simulink model "controller_dev_sg_RCP"  (R2018b)
settings: configuration reference "Active" (kept outside this file)
model workspace (MAT data in the model file):
  m = 1000
undefined symbols (not defined in the file or in its folder): C, tS, TUMHealthStatus, TUMVehicleState
libraries: xpcrtudplib x6, simulink x6, canmsglib x6, etargetslib x5, misc x4, speedgoatlib_IO614 x3, slrtlib x2
(part 3 of 3)

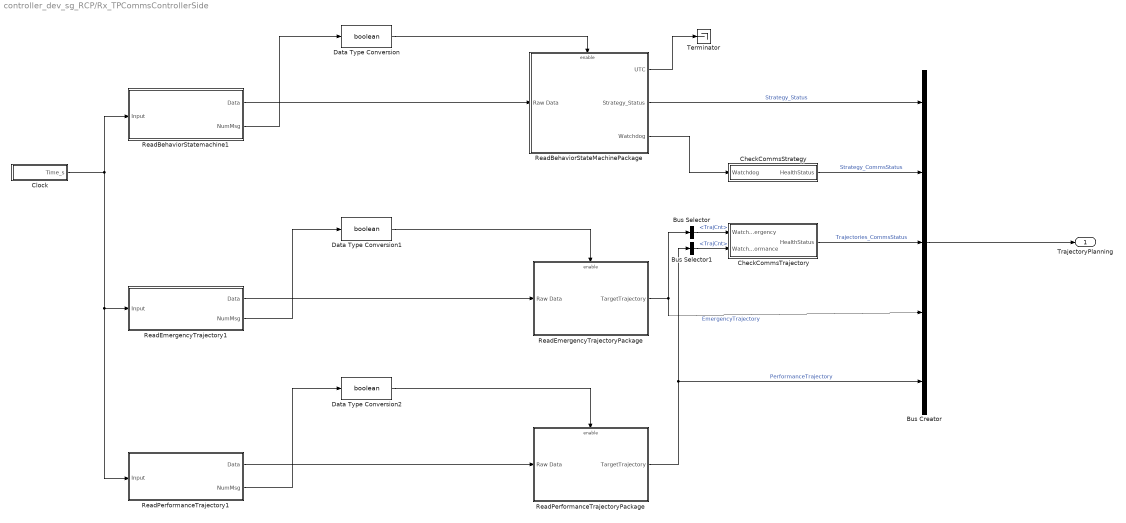
== system controller_dev_sg_RCP/Rx_TPCommsControllerSide ==
  Bus Creator : BusCreator  Inputs=5
  Bus Selector : BusSelector  OutputSignals=TrajCnt
  Bus Selector1 : BusSelector  OutputSignals=TrajCnt
  CheckCommsStrategy : Subsystem
  CheckCommsTrajectory : Subsystem
  Clock : Subsystem
  Data Type Conversion : DataTypeConversion  OutDataTypeStr=boolean
  Data Type Conversion1 : DataTypeConversion  OutDataTypeStr=boolean
  Data Type Conversion2 : DataTypeConversion  OutDataTypeStr=boolean
  ReadBehaviorStateMachinePackage : Subsystem  Priority=1000
  ReadBehaviorStatemachine1 : Subsystem  Priority=1
  ReadEmergencyTrajectory1 : Subsystem  Priority=1000
  ReadEmergencyTrajectoryPackage : Subsystem  Priority=1000
  ReadPerformanceTrajectory1 : Subsystem  Priority=1000
  ReadPerformanceTrajectoryPackage : Subsystem  Priority=1000
  Terminator : Terminator
  TrajectoryPlanning : Outport  OutDataTypeStr=Bus: TrajectoryPlanning  BusOutputAsStruct=on
  wires:
  ReadBehaviorStateMachinePackage/1(UTC) -> Terminator/1
  ReadPerformanceTrajectoryPackage/1(TargetTrajectory) -> Bus Selector1/1, Bus Creator/5  "PerformanceTrajectory"
  Clock/1(Time_s) -> ReadPerformanceTrajectory1/1(Input), ReadEmergencyTrajectory1/1(Input), ReadBehaviorStatemachine1/1(Input)
  CheckCommsTrajectory/1(HealthStatus) -> Bus Creator/3  "Trajectories_CommsStatus"
  ReadBehaviorStateMachinePackage/2(Strategy_Status) -> Bus Creator/1  "Strategy_Status"
  CheckCommsStrategy/1(HealthStatus) -> Bus Creator/2  "Strategy_CommsStatus"
  ReadEmergencyTrajectoryPackage/1(TargetTrajectory) -> Bus Selector/1, Bus Creator/4  "EmergencyTrajectory"
  Bus Selector/1 -> CheckCommsTrajectory/1(WatchdogEmergency)  "<TrajCnt>"
  Bus Selector1/1 -> CheckCommsTrajectory/2(WatchdogPerformance)  "<TrajCnt>"
  ReadBehaviorStateMachinePackage/3(Watchdog) -> CheckCommsStrategy/1(Watchdog)
  ReadEmergencyTrajectory1/2(NumMsg) -> Data Type Conversion1/1
  ReadPerformanceTrajectory1/2(NumMsg) -> Data Type Conversion2/1
  ReadBehaviorStatemachine1/2(NumMsg) -> Data Type Conversion/1
  ReadBehaviorStatemachine1/1(Data) -> ReadBehaviorStateMachinePackage/1(Raw Data)
  Data Type Conversion/1 -> ReadBehaviorStateMachinePackage/Enable
  Bus Creator/1 -> TrajectoryPlanning/1
  Data Type Conversion1/1 -> ReadEmergencyTrajectoryPackage/Enable
  ReadEmergencyTrajectory1/1(Data) -> ReadEmergencyTrajectoryPackage/1(Raw Data)
  ReadPerformanceTrajectory1/1(Data) -> ReadPerformanceTrajectoryPackage/1(Raw Data)
  Data Type Conversion2/1 -> ReadPerformanceTrajectoryPackage/Enable

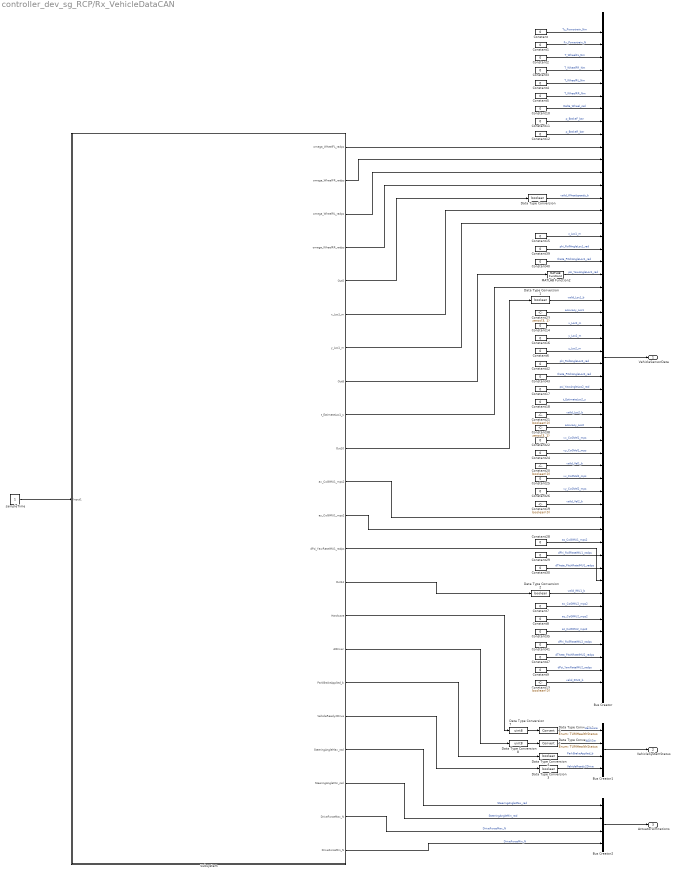
== system controller_dev_sg_RCP/Rx_VehicleDataCAN ==
  Bus Creator : BusCreator  Inputs=52  OutDataTypeStr=Bus: VehicleSensorData
  Bus Creator1 : BusCreator  Inputs=4  OutDataTypeStr=Bus: VehicleSystemStatus
  Bus Creator2 : BusCreator  Inputs=4  OutDataTypeStr=Bus: ActuatorLimitations
  Constant{,1..12,14..18,22,24..26,28..30,35,39..43,47} (32 alike) : Constant  Value=0
  Constant{13,19..21} (4 alike) : Constant  Value=boolean(0)
  Constant23 : Constant  Value=zeros(3, 1)
  Constant38 : Constant  Value=zeros(3, 1)
  Data Type Conversion{,1..4} (5 alike) : DataTypeConversion  OutDataTypeStr=boolean
  Data Type Conversion5 : DataTypeConversion  OutDataTypeStr=Enum: TUMHealthStatus
  Data Type Conversion6 : DataTypeConversion  OutDataTypeStr=Enum: TUMHealthStatus
  Data Type Conversion7 : DataTypeConversion  OutDataTypeStr=uint8
  Data Type Conversion8 : DataTypeConversion  OutDataTypeStr=uint8
  MATLAB Function2 : misc/MATLAB Function2  SystemSampleTime=-1
  Subsystem : Subsystem
  sampleTime : Constant  SampleTime=tS
  VehicleSensorData : Outport  OutDataTypeStr=Bus: VehicleSensorData
  VehicleSystemStatus : Outport  Port=2  OutDataTypeStr=Bus: VehicleSystemStatus
  ActuatorLImitations : Outport  Port=3  OutDataTypeStr=Bus: ActuatorLimitations
  wires:
  Constant30/1 -> Bus Creator/43  "dTheta_PitchRateIMU1_radps"
  Constant12/1 -> Bus Creator/9  "p_BrakeR_bar"
  Constant5/1 -> Bus Creator/6  "T_WheelRR_Nm"
  Constant1/1 -> Bus Creator/2  "Fx_Powertrain_N"
  Constant19/1 -> Bus Creator/38  "valid_Vel2_b"
  Constant7/1 -> Bus Creator/46  "ax_CoGIMU2_mps2"
  Constant11/1 -> Bus Creator/8  "p_BrakeF_bar"
  Bus Creator/1 -> VehicleSensorData/1
  Constant21/1 -> Bus Creator/31  "valid_Loc2_b"
  Constant/1 -> Bus Creator/1  "Tz_Powertrain_Nm"
  Constant25/1 -> Bus Creator/36  "vx_CoGVel2_mps"
  Constant38/1 -> Bus Creator/32  "accuracy_Loc2"
  Constant8/1 -> Bus Creator/47  "ay_CoGIMU2_mps2"
  Constant3/1 -> Bus Creator/4  "T_WheelFR_Nm"
  Constant10/1 -> Bus Creator/7  "Delta_Wheel_rad"
  Constant14/1 -> Bus Creator/24  "x_Loc2_m"
  Constant40/1 -> Bus Creator/19  "theta_PitchAngleLoc1_rad"
  Constant23/1 -> Bus Creator/23  "accuracy_Loc1"
  Constant4/1 -> Bus Creator/5  "T_WheelRL_Nm"
  Constant28/1 -> Bus Creator/41  "az_CoGIMU1_mps2"
  Constant20/1 -> Bus Creator/35  "valid_Vel1_b"
  Constant6/1 -> Bus Creator/26  "z_Loc2_m"
  Constant2/1 -> Bus Creator/3  "T_WheelFL_Nm"
  Constant39/1 -> Bus Creator/18  "phi_RollAngleLoc1_rad"
  Constant15/1 -> Bus Creator/17  "z_Loc1_m"
  Constant26/1 -> Bus Creator/37  "vy_CoGVel2_mps"
  Constant16/1 -> Bus Creator/25  "y_Loc2_m"
  MATLAB Function2/1 -> Bus Creator/20  "psi_YawAngleLoc1_rad"
  Constant42/1 -> Bus Creator/27  "phi_RollAngleLoc2_rad"
  Constant9/1 -> Bus Creator/51  "dPsi_YawRateIMU2_radps"
  Constant17/1 -> Bus Creator/29  "psi_YawAngleLoc2_rad"
  Constant24/1 -> Bus Creator/34  "vy_CoGVel1_mps"
  Constant13/1 -> Bus Creator/52  "valid_IMU2_b"
  Constant29/1 -> Bus Creator/42  "dPhi_RollRateIMU1_radps"
  Constant22/1 -> Bus Creator/33  "vx_CoGVel1_mps"
  Constant18/1 -> Bus Creator/30  "t_EstimateLoc2_s"
  Constant43/1 -> Bus Creator/28  "theta_PitchAngleLoc2_rad"
  Constant47/1 -> Bus Creator/50  "dTheta_PitchRateIMU2_radps"
  Constant41/1 -> Bus Creator/49  "dPhi_RollRateIMU2_radps"
  Constant35/1 -> Bus Creator/48  "az_CoGIMU2_mps2"
  Bus Creator1/1 -> VehicleSystemStatus/1
  Bus Creator2/1 -> ActuatorLImitations/1
  Data Type Conversion/1 -> Bus Creator/14  "valid_Wheelspeeds_b"
  Data Type Conversion1/1 -> Bus Creator/22  "valid_Loc1_b"
  Data Type Conversion2/1 -> Bus Creator/45  "valid_IMU1_b"
  Data Type Conversion3/1 -> Bus Creator1/4  "VehicleReady2Drive"
  Data Type Conversion4/1 -> Bus Creator1/3  "ParkBrakeApplied_b"
  Data Type Conversion5/1 -> Bus Creator1/2  "AIDriver"
  Data Type Conversion6/1 -> Bus Creator1/1  "Hardware"
  Data Type Conversion7/1 -> Data Type Conversion6/1
  Data Type Conversion8/1 -> Data Type Conversion5/1
  Subsystem/1(omega_WheelFL_radps) -> Bus Creator/10
  Subsystem/2(omega_WheelFR_radps) -> Bus Creator/11
  Subsystem/3(omega_WheelRL_radps) -> Bus Creator/12
  Subsystem/4(omega_WheelRR_radps) -> Bus Creator/13
  Subsystem/5(Out5) -> Data Type Conversion/1
  Subsystem/6(x_Loc1_m) -> Bus Creator/15
  Subsystem/7(y_Loc1_m) -> Bus Creator/16
  Subsystem/8(Out8) -> MATLAB Function2/1
  Subsystem/9(t_EstimateLoc1_s) -> Bus Creator/21
  Subsystem/10(Out10) -> Data Type Conversion1/1
  Subsystem/11(ax_CoGIMU1_mps2) -> Bus Creator/39
  Subsystem/12(ay_CoGIMU1_mps2) -> Bus Creator/40
  Subsystem/13(dPsi_YawRateIMU1_radps) -> Bus Creator/44
  Subsystem/14(Out14) -> Data Type Conversion2/1
  Subsystem/15(Hardware) -> Data Type Conversion7/1
  Subsystem/16(AIDriver) -> Data Type Conversion8/1
  Subsystem/17(ParkBrakeApplied_b) -> Data Type Conversion4/1
  Subsystem/18(VehicleReady2Drive) -> Data Type Conversion3/1
  sampleTime/1 -> Subsystem/1(Input1)
  Subsystem/22(DriveForceMin_N) -> Bus Creator2/4  "DriveForceMin_N"
  Subsystem/19(SteeringAngleMax_rad) -> Bus Creator2/1  "SteeringAngleMax_rad"
  Subsystem/20(SteeringAngleMin_rad) -> Bus Creator2/2  "SteeringAngleMin_rad"
  Subsystem/21(DriveForceMax_N) -> Bus Creator2/3  "DriveForceMax_N"

== system controller_dev_sg_RCP/Tx_TPCommsControllerSide ==
  VehicleDynamicState : Inport
  TrajPlannerSend : Inport  Port=2
  DebugData : Inport  Port=3
  BehaviorStatemachine : Subsystem
  Digital Clock : DigitalClock  SampleTime=-1
  SendToBehaviorStatemachine1 : Subsystem
  SendToTrajectoryGeneration1 : Subsystem
  TrajectoryGeneration : Subsystem
  wires:
  DebugData/1 -> BehaviorStatemachine/2(DebugData)
  TrajPlannerSend/1 -> TrajectoryGeneration/1(TrajPlannerSend), BehaviorStatemachine/1(TrajPlannerSend)
  VehicleDynamicState/1 -> TrajectoryGeneration/2(VehicleDynamicState)
  Digital Clock/1 -> TrajectoryGeneration/3(Time_s)
  BehaviorStatemachine/2(BSM_Package) -> SendToBehaviorStatemachine1/1(Data)  "BSM_Package"
  TrajectoryGeneration/2(TG_Package) -> SendToTrajectoryGeneration1/1(Data)
  TrajectoryGeneration/1(TG_ActivateSend) -> SendToTrajectoryGeneration1/Enable  "TG_ActivateSend"
  BehaviorStatemachine/1(BSM_ActivateSend) -> SendToBehaviorStatemachine1/Enable  "BSM_ActivateSend"

== system controller_dev_sg_RCP/Tx_VehicleControlCAN ==
  SteeringAngleAtWheel_rad : Inport
  TractionForceSummedAtWheels_N : Inport  Port=2
  "CAN Pack " : canmsglib/CAN Pack  MsgList=(none)  MsgName=CAN Msg  MsgIDType=Standard (11-bit identifier)  MsgIdentifier=24  MsgLength=8  SignalInfo=SteeringAngleAtWheel_rad$0$24$1$1$1$0$0.000001$0$-Inf$Inf$#TractionForceSummedAtWheels_N$24$24$1$1$1$0$0.01$0$-Inf$Inf$#  NSignals=2  StartBits=str2num('[int32(0);int32(24)]')  SignalSizes=str2num('[int32(24);int32(24)]')  ByteOrders=str2num('[int32(1);int32(1)]')  DataTypes=str2num('[int32(1);int32(1)]')  MultiplexTypes=str2num('[int32(1);int32(1)]')  MultiplexValues=str2num('[double(0);double(0)]')  Factors=str2num('[double(0.000001);double(0.01)]')  Offsets=str2num('[double(0);double(0)]')  Minimums=str2num('[double(-Inf);double(-Inf)]')  Maximums=str2num('[double(Inf);double(Inf)]')  Remote=off  ApplyMinMax=off  BusOutput=off
      settings: SourceProductName=Simulink Real-Time  DataFormat=manually specified signals
  CAN Write : speedgoatlib_IO614/CAN/CAN Write  id=1  sampleTime=-1  portSelection=2  messageType=CAN  enaStatusPort=off  protl=IO614  ptIdx=1  isFDMod=0
      settings: SourceProductName=Simulink Real-Time: Speedgoat Library
  wires:
  "CAN Pack "/1 -> CAN Write/1
  TractionForceSummedAtWheels_N/1 -> "CAN Pack "/2
  SteeringAngleAtWheel_rad/1 -> "CAN Pack "/1

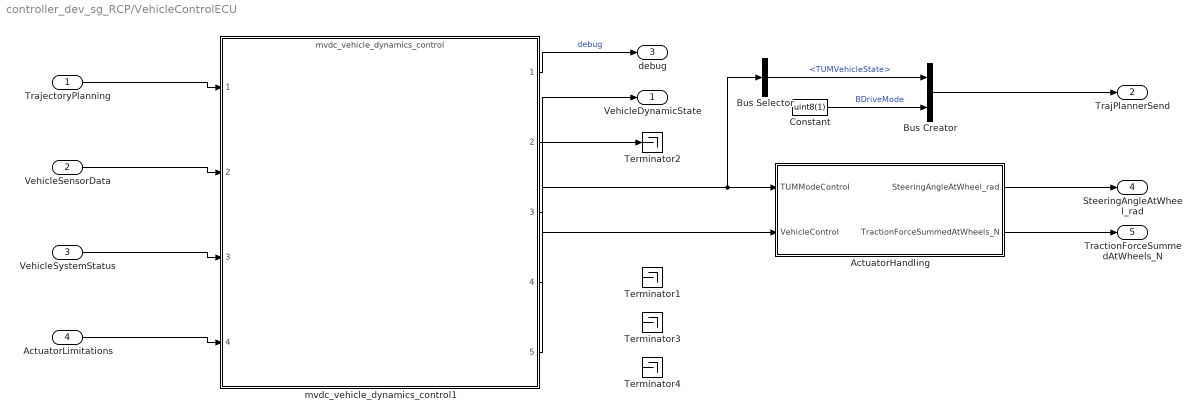
== system controller_dev_sg_RCP/VehicleControlECU ==
  TrajectoryPlanning : Inport
  VehicleSensorData : Inport  Port=2
  VehicleSystemStatus : Inport  Port=3
  ActuatorLimitations : Inport  Port=4
  ActuatorHandling : Subsystem
  Bus Creator : BusCreator  Inputs=2
  Bus Selector : BusSelector  OutputSignals=TUMVehicleState
  Constant : Constant  Value=uint8(1)
  Terminator{1..4} (4 alike) : Terminator
  mvdc_vehicle_dynamics_control1 : ModelReference  ModelNameDialog=mvdc_vehicle_dynamics_control  SimulationMode=Normal  ModelReferenceVersion=1.767
  VehicleDynamicState : Outport
  TrajPlannerSend : Outport  Port=2
  debug : Outport  Port=3
  SteeringAngleAtWheel_rad : Outport  Port=4
  TractionForceSummedAtWheels_N : Outport  Port=5
  wires:
  mvdc_vehicle_dynamics_control1/1 -> debug/1  "debug"
  VehicleSystemStatus/1 -> mvdc_vehicle_dynamics_control1/3
  ActuatorLimitations/1 -> mvdc_vehicle_dynamics_control1/4
  VehicleSensorData/1 -> mvdc_vehicle_dynamics_control1/2
  mvdc_vehicle_dynamics_control1/5 -> ActuatorHandling/2(VehicleControl)
  mvdc_vehicle_dynamics_control1/4 -> Bus Selector/1, ActuatorHandling/1(TUMModeControl)
  ? -> Terminator1/1
  mvdc_vehicle_dynamics_control1/3 -> Terminator2/1
  mvdc_vehicle_dynamics_control1/2 -> VehicleDynamicState/1
  ActuatorHandling/2(TractionForceSummedAtWheels_N) -> TractionForceSummedAtWheels_N/1
  ActuatorHandling/1(SteeringAngleAtWheel_rad) -> SteeringAngleAtWheel_rad/1
  ? -> Terminator3/1
  ? -> Terminator4/1
  Bus Selector/1 -> Bus Creator/1  "<TUMVehicleState>"
  Constant/1 -> Bus Creator/2  "BDriveMode"
  Bus Creator/1 -> TrajPlannerSend/1
  TrajectoryPlanning/1 -> mvdc_vehicle_dynamics_control1/1

== system controller_dev_sg_RCP/Rx_TPCommsControllerSide/CheckCommsStrategy ==
  Watchdog : Inport
  CheckComms : misc/CheckComms  timeout_s=tPX2CommsTimeout  tS=tS
  Constant1 : Constant  Value=TUMHealthStatus.ERROR  OutDataTypeStr=Enum: TUMHealthStatus
  Constant2 : Constant  Value=TUMHealthStatus.OK  OutDataTypeStr=Enum: TUMHealthStatus
  Switch1 : Switch  Criteria=u2 > Threshold
  HealthStatus : Outport
  wires:
  CheckComms/1 -> Switch1/2
  Constant2/1 -> Switch1/1
  Switch1/1 -> HealthStatus/1  "Strategy_CommsStatus"
  Constant1/1 -> Switch1/3
  Watchdog/1 -> CheckComms/1

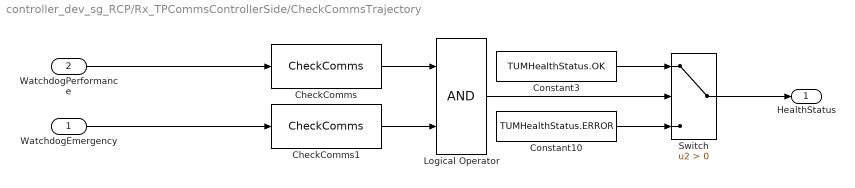
== system controller_dev_sg_RCP/Rx_TPCommsControllerSide/CheckCommsTrajectory ==
  WatchdogEmergency : Inport
  WatchdogPerformance : Inport  Port=2
  CheckComms : misc/CheckComms  timeout_s=tPX2CommsTimeout  tS=tS
  CheckComms1 : misc/CheckComms  timeout_s=tPX2CommsTimeout  tS=tS
  Constant10 : Constant  Value=TUMHealthStatus.ERROR  OutDataTypeStr=Enum: TUMHealthStatus  SampleTime=-1
  Constant3 : Constant  Value=TUMHealthStatus.OK  OutDataTypeStr=Enum: TUMHealthStatus  SampleTime=-1
  Logical Operator : Logic  AllPortsSameDT=off  OutDataTypeStr=boolean
  Switch : Switch  Criteria=u2 > Threshold
  HealthStatus : Outport
  wires:
  Constant10/1 -> Switch/3
  Logical Operator/1 -> Switch/2
  CheckComms/1 -> Logical Operator/1
  CheckComms1/1 -> Logical Operator/2
  Constant3/1 -> Switch/1
  Switch/1 -> HealthStatus/1
  WatchdogEmergency/1 -> CheckComms1/1
  WatchdogPerformance/1 -> CheckComms/1

== system controller_dev_sg_RCP/Rx_TPCommsControllerSide/Clock ==
  Counter Free-Running : simulink/Sources/Counter Free-Running  NumBits=32  tsamp=tS
  Data Type Conversion : DataTypeConversion  OutDataTypeStr=double  SaturateOnIntegerOverflow=on
  Gain : Gain  Gain=tS
  Time_s : Outport
  wires:
  Counter Free-Running/1 -> Data Type Conversion/1
  Gain/1 -> Time_s/1
  Data Type Conversion/1 -> Gain/1

== system controller_dev_sg_RCP/Rx_TPCommsControllerSide/ReadBehaviorStateMachinePackage ==
  Raw Data : Inport
  Enable : EnablePort
  Byte Unpack : etargetslib/Byte Unpack  dimensions={[1], [1], [1]}  datatypes={'uint16', 'uint16', 'uint32'}  byteAlign=1
  Data Type Conversion : DataTypeConversion  OutDataTypeStr=Enum: TUMStrategyState  SaturateOnIntegerOverflow=on
  UTC : Outport
  Strategy_Status : Outport  Port=2  OutDataTypeStr=Enum: TUMStrategyState
  Watchdog : Outport  Port=3
  wires:
  Byte Unpack/1 -> Data Type Conversion/1
  Data Type Conversion/1 -> Strategy_Status/1
  Byte Unpack/2 -> Watchdog/1
  Raw Data/1 -> Byte Unpack/1
  Byte Unpack/3 -> UTC/1

== system controller_dev_sg_RCP/Rx_TPCommsControllerSide/ReadBehaviorStatemachine1 ==
  Input : Inport
  Compare To Constant : simulink/Logic and Bit Operations/Compare To Constant  Priority=1  relop===  const=8  OutDataTypeStr=boolean
  Min. do-while count : Constant  OutDataTypeStr=int8  SampleTime=-1
  Subtrat : Sum  Inputs=+-
  Terminator : Terminator
  UDP Receive : xpcrtudplib/UDP Receive  ipAddressVal=10.0.0.1  localPort=BehaviorStatemachineRcv_Port  rcvWidth=8  rcvFmAny=off  fmAddress=10.0.0.2  rcvMulticast=off  multicastAddress={}  maxUDPQueue=8  sampleTime=-1
      settings: SourceProductName=Simulink Real-Time
  While Iterator : WhileIterator  WhileBlockType=do-while  ShowIterationPort=on  OutputDataType=int16
  Data : Outport
  NumMsg : Outport  Port=2
  wires:
  Compare To Constant/1 -> While Iterator/1
  UDP Receive/2 -> Compare To Constant/1
  While Iterator/1 -> Subtrat/1
  Min. do-while count/1 -> Subtrat/2
  UDP Receive/1 -> Data/1
  Subtrat/1 -> NumMsg/1  "num msgs this timestep"
  Input/1 -> Terminator/1

== system controller_dev_sg_RCP/Rx_TPCommsControllerSide/ReadEmergencyTrajectory1 ==
  Input : Inport
  Compare To Constant : simulink/Logic and Bit Operations/Compare To Constant  relop===  const=4*7*50+2*4  OutDataTypeStr=boolean
  Min. do-while count : Constant  OutDataTypeStr=int8  SampleTime=-1
  Subtrat : Sum  Inputs=+-
  Terminator : Terminator
  UDP Receive : xpcrtudplib/UDP Receive  ipAddressVal=10.0.0.1  localPort=EmergencyPathRcv_Port  rcvWidth=4*7*50+2*4  rcvFmAny=off  fmAddress=10.0.0.2  rcvMulticast=off  multicastAddress={}  maxUDPQueue=8  sampleTime=-1
      settings: SourceProductName=Simulink Real-Time
  While Iterator : WhileIterator  WhileBlockType=do-while  ShowIterationPort=on  OutputDataType=int16
  Data : Outport
  NumMsg : Outport  Port=2
  wires:
  UDP Receive/2 -> Compare To Constant/1
  While Iterator/1 -> Subtrat/1
  Min. do-while count/1 -> Subtrat/2
  UDP Receive/1 -> Data/1
  Compare To Constant/1 -> While Iterator/1
  Subtrat/1 -> NumMsg/1  "num msgs this timestep"
  Input/1 -> Terminator/1

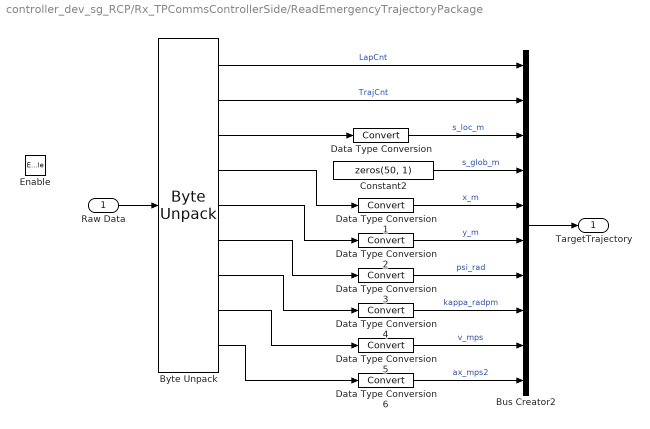
== system controller_dev_sg_RCP/Rx_TPCommsControllerSide/ReadEmergencyTrajectoryPackage ==
  Raw Data : Inport
  Enable : EnablePort
  Bus Creator2 : BusCreator  Inputs=10  OutDataTypeStr=Bus: Trajectory
      settings: InheritFromInputs=off
  Byte Unpack : etargetslib/Byte Unpack  dimensions={[1], [1], [50], [50], [50], [50], [50], [50],[50]}  datatypes={'uint32', 'uint32', 'single', 'single', 'single', 'single', 'single', 'single', 'single'}  byteAlign=1
  Constant2 : Constant  Value=zeros(50, 1)
  Data Type Conversion{,1..6} (7 alike) : DataTypeConversion
  TargetTrajectory : Outport  OutDataTypeStr=Bus: Trajectory
  wires:
  Byte Unpack/1 -> Bus Creator2/1  "LapCnt"
  Byte Unpack/2 -> Bus Creator2/2  "TrajCnt"
  Bus Creator2/1 -> TargetTrajectory/1
  Raw Data/1 -> Byte Unpack/1
  Byte Unpack/3 -> Data Type Conversion/1
  Byte Unpack/4 -> Data Type Conversion1/1
  Constant2/1 -> Bus Creator2/4  "s_glob_m"
  Data Type Conversion/1 -> Bus Creator2/3  "s_loc_m"
  Data Type Conversion1/1 -> Bus Creator2/5  "x_m"
  Data Type Conversion2/1 -> Bus Creator2/6  "y_m"
  Byte Unpack/5 -> Data Type Conversion2/1
  Data Type Conversion3/1 -> Bus Creator2/7  "psi_rad"
  Data Type Conversion4/1 -> Bus Creator2/8  "kappa_radpm"
  Data Type Conversion5/1 -> Bus Creator2/9  "v_mps"
  Data Type Conversion6/1 -> Bus Creator2/10  "ax_mps2"
  Byte Unpack/6 -> Data Type Conversion3/1
  Byte Unpack/7 -> Data Type Conversion4/1
  Byte Unpack/8 -> Data Type Conversion5/1
  Byte Unpack/9 -> Data Type Conversion6/1

== system controller_dev_sg_RCP/Rx_TPCommsControllerSide/ReadPerformanceTrajectory1 ==
  Input : Inport
  Compare To Constant : simulink/Logic and Bit Operations/Compare To Constant  relop===  const=4*7*50+2*4  OutDataTypeStr=boolean
  Min. do-while count : Constant  OutDataTypeStr=int8  SampleTime=-1
  Subtrat : Sum  Inputs=+-
  Terminator : Terminator
  UDP Receive : xpcrtudplib/UDP Receive  ipAddressVal=10.0.0.1  localPort=PerformanceTrajectoryRcv_Port  rcvWidth=4*7*50+2*4  rcvFmAny=off  fmAddress=10.0.0.2  rcvMulticast=off  multicastAddress={}  maxUDPQueue=8  sampleTime=-1
      settings: SourceProductName=Simulink Real-Time
  While Iterator : WhileIterator  WhileBlockType=do-while  ShowIterationPort=on  OutputDataType=int16
  Data : Outport
  NumMsg : Outport  Port=2
  wires:
  Compare To Constant/1 -> While Iterator/1
  UDP Receive/2 -> Compare To Constant/1
  UDP Receive/1 -> Data/1
  While Iterator/1 -> Subtrat/1
  Min. do-while count/1 -> Subtrat/2
  Subtrat/1 -> NumMsg/1  "num msgs this timestep"
  Input/1 -> Terminator/1

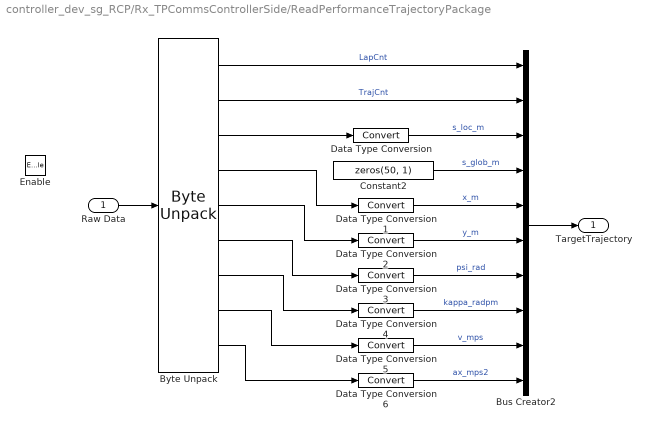
== system controller_dev_sg_RCP/Rx_TPCommsControllerSide/ReadPerformanceTrajectoryPackage ==
  Raw Data : Inport
  Enable : EnablePort
  Bus Creator2 : BusCreator  Inputs=10  OutDataTypeStr=Bus: Trajectory
      settings: InheritFromInputs=off
  Byte Unpack : etargetslib/Byte Unpack  dimensions={[1], [1], [50], [50], [50], [50], [50], [50],[50]}  datatypes={'uint32', 'uint32', 'single', 'single', 'single', 'single', 'single', 'single', 'single'}  byteAlign=1
  Constant2 : Constant  Value=zeros(50, 1)
  Data Type Conversion{,1..6} (7 alike) : DataTypeConversion
  TargetTrajectory : Outport  OutDataTypeStr=Bus: Trajectory
  wires:
  Byte Unpack/1 -> Bus Creator2/1  "LapCnt"
  Byte Unpack/2 -> Bus Creator2/2  "TrajCnt"
  Bus Creator2/1 -> TargetTrajectory/1
  Raw Data/1 -> Byte Unpack/1
  Byte Unpack/3 -> Data Type Conversion/1
  Byte Unpack/4 -> Data Type Conversion1/1
  Constant2/1 -> Bus Creator2/4  "s_glob_m"
  Data Type Conversion/1 -> Bus Creator2/3  "s_loc_m"
  Data Type Conversion1/1 -> Bus Creator2/5  "x_m"
  Data Type Conversion2/1 -> Bus Creator2/6  "y_m"
  Byte Unpack/5 -> Data Type Conversion2/1
  Data Type Conversion3/1 -> Bus Creator2/7  "psi_rad"
  Data Type Conversion4/1 -> Bus Creator2/8  "kappa_radpm"
  Data Type Conversion5/1 -> Bus Creator2/9  "v_mps"
  Data Type Conversion6/1 -> Bus Creator2/10  "ax_mps2"
  Byte Unpack/6 -> Data Type Conversion3/1
  Byte Unpack/7 -> Data Type Conversion4/1
  Byte Unpack/8 -> Data Type Conversion5/1
  Byte Unpack/9 -> Data Type Conversion6/1

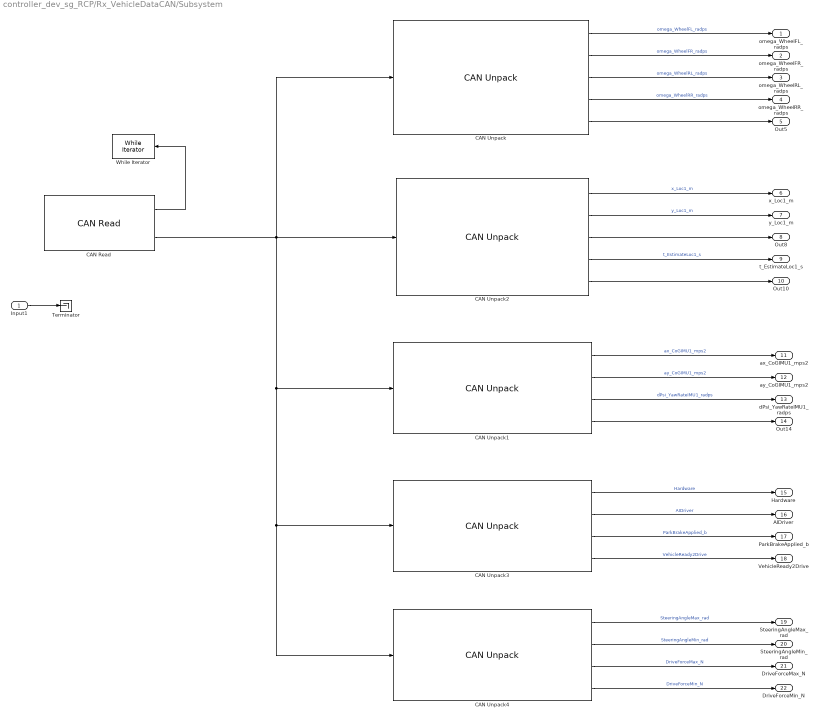
== system controller_dev_sg_RCP/Rx_VehicleDataCAN/Subsystem ==
  Input1 : Inport
  CAN Read : speedgoatlib_IO614/CAN/CAN Read  id=1  sampleTime=-1  portSelection=1  messageType=CAN  protl=IO614  ptIdx=0  isFDMod=0
      settings: SourceProductName=Simulink Real-Time: Speedgoat Library
  CAN Unpack : canmsglib/CAN Unpack  MsgList=(none)  MsgName=CAN Msg  MsgIDType=Standard (11-bit identifier)  MsgIdentifier=768  MsgLength=8  SignalInfo=omega_WheelFL_radps$0$15$1$1$1$0$0.1$0$-Inf$Inf$#omega_WheelFR_radps$15$15$1$1$1$0$0.1$0$-Inf$Inf$#omega_WheelRL_radps$30$15$1$1$1$0$0.1$0$-Inf$Inf$#omega_WheelRR_radps$45$15$1$1$1$0$0.1$0$-Inf$Inf$#valid_Wheelspeeds_b$60$4$1$1$1$0$1$0$-Inf$Inf$#  NSignals=5  IDPort=off  TimestampPort=off  ErrorPort=off  RemotePort=off  LengthPort=off  StatusPort=off  StartBits=str2num('[int32(0);int32(15);int32(30);int32(45);int32(60)]')  SignalSizes=str2num('[int32(15);int32(15);int32(15);int32(15);int32(4)]')  ByteOrders=str2num('[int32(1);int32(1);int32(1);int32(1);int32(1)]')  DataTypes=str2num('[int32(1);int32(1);int32(1);int32(1);int32(1)]')  MultiplexTypes=str2num('[int32(1);int32(1);int32(1);int32(1);int32(1)]')  MultiplexValues=str2num('[double(0);double(0);double(0);double(0);double(0)]')  Factors=str2num('[double(0.1);double(0.1);double(0.1);double(0.1);double(1)]')  Offsets=str2num('[double(0);double(0);double(0);double(0);double(0)]')  Minimums=str2num('[double(-Inf);double(-Inf);double(-Inf);double(-Inf);double(-Inf)]')  Maximums=str2num('[double(Inf);double(Inf);double(Inf);double(Inf);double(Inf)]')  ApplyMinMax=off
      settings: SourceProductName=Simulink Real-Time
  CAN Unpack1 : canmsglib/CAN Unpack  MsgList=(none)  MsgName=CAN Msg  MsgIDType=Standard (11-bit identifier)  MsgIdentifier=48  MsgLength=8  SignalInfo=ax_CoGIMU1_mps2$0$16$1$1$1$0$0.001$0$-Inf$Inf$#ay_CoGIMU1_mps2$16$16$1$1$1$0$0.001$0$-Inf$Inf$#dPsi_YawRateIMU1_radps$32$16$1$1$1$0$0.0001$0$-Inf$Inf$#valid_IMU1_b$48$16$1$1$1$0$1$0$-Inf$Inf$#  NSignals=4  IDPort=off  TimestampPort=off  ErrorPort=off  RemotePort=off  LengthPort=off  StatusPort=off  StartBits=str2num('[int32(0);int32(16);int32(32);int32(48)]')  SignalSizes=str2num('[int32(16);int32(16);int32(16);int32(16)]')  ByteOrders=str2num('[int32(1);int32(1);int32(1);int32(1)]')  DataTypes=str2num('[int32(1);int32(1);int32(1);int32(1)]')  MultiplexTypes=str2num('[int32(1);int32(1);int32(1);int32(1)]')  MultiplexValues=str2num('[double(0);double(0);double(0);double(0)]')  Factors=str2num('[double(0.001);double(0.001);double(0.0001);double(1)]')  Offsets=str2num('[double(0);double(0);double(0);double(0)]')  Minimums=str2num('[double(-Inf);double(-Inf);double(-Inf);double(-Inf)]')  Maximums=str2num('[double(Inf);double(Inf);double(Inf);double(Inf)]')  ApplyMinMax=off
      settings: SourceProductName=Simulink Real-Time
  CAN Unpack2 : canmsglib/CAN Unpack  MsgList=(none)  MsgName=CAN Msg  MsgIDType=Standard (11-bit identifier)  MsgIdentifier=192  MsgLength=8  SignalInfo=x_Loc1_m$0$15$1$1$1$0$0.05$0$-Inf$Inf$#y_Loc1_m$15$15$1$1$1$0$0.05$0$-Inf$Inf$#psi_YawAngleLoc1_rad$30$15$1$1$1$0$0.001$0$-Inf$Inf$#t_EstimateLoc1_s$45$15$1$1$1$0$0.001$0$-Inf$Inf$#valid_Loc1_b$60$4$1$1$1$0$1$0$-Inf$Inf$#  NSignals=5  IDPort=off  TimestampPort=off  ErrorPort=off  RemotePort=off  LengthPort=off  StatusPort=off  StartBits=str2num('[int32(0);int32(15);int32(30);int32(45);int32(60)]')  SignalSizes=str2num('[int32(15);int32(15);int32(15);int32(15);int32(4)]')  ByteOrders=str2num('[int32(1);int32(1);int32(1);int32(1);int32(1)]')  DataTypes=str2num('[int32(1);int32(1);int32(1);int32(1);int32(1)]')  MultiplexTypes=str2num('[int32(1);int32(1);int32(1);int32(1);int32(1)]')  MultiplexValues=str2num('[double(0);double(0);double(0);double(0);double(0)]')  Factors=str2num('[double(0.05);double(0.05);double(0.001);double(0.001);double(1)]')  Offsets=str2num('[double(0);double(0);double(0);double(0);double(0)]')  Minimums=str2num('[double(-Inf);double(-Inf);double(-Inf);double(-Inf);double(-Inf)]')  Maximums=str2num('[double(Inf);double(Inf);double(Inf);double(Inf);double(Inf)]')  ApplyMinMax=off
      settings: SourceProductName=Simulink Real-Time
  CAN Unpack3 : canmsglib/CAN Unpack  MsgList=(none)  MsgName=CAN Msg  MsgIDType=Standard (11-bit identifier)  MsgIdentifier=12  MsgLength=8  SignalInfo=Hardware$0$12$1$2$1$0$1$0$-Inf$Inf$#AIDriver$12$12$1$2$1$0$1$0$-Inf$Inf$#ParkBrakeApplied_b$24$12$1$1$1$0$1$0$-Inf$Inf$#VehicleReady2Drive$36$12$1$1$1$0$1$0$-Inf$Inf$#  NSignals=4  IDPort=off  TimestampPort=off  ErrorPort=off  RemotePort=off  LengthPort=off  StatusPort=off  StartBits=str2num('[int32(0);int32(12);int32(24);int32(36)]')  SignalSizes=str2num('[int32(12);int32(12);int32(12);int32(12)]')  ByteOrders=str2num('[int32(1);int32(1);int32(1);int32(1)]')  DataTypes=str2num('[int32(2);int32(2);int32(1);int32(1)]')  MultiplexTypes=str2num('[int32(1);int32(1);int32(1);int32(1)]')  MultiplexValues=str2num('[double(0);double(0);double(0);double(0)]')  Factors=str2num('[double(1);double(1);double(1);double(1)]')  Offsets=str2num('[double(0);double(0);double(0);double(0)]')  Minimums=str2num('[double(-Inf);double(-Inf);double(-Inf);double(-Inf)]')  Maximums=str2num('[double(Inf);double(Inf);double(Inf);double(Inf)]')  ApplyMinMax=off
      settings: SourceProductName=Simulink Real-Time
  CAN Unpack4 : canmsglib/CAN Unpack  MsgList=(none)  MsgName=CAN Msg  MsgIDType=Standard (11-bit identifier)  MsgIdentifier=170  MsgLength=8  SignalInfo=SteeringAngleMax_rad$0$16$1$1$1$0$0.001$0$-Inf$Inf$#SteeringAngleMin_rad$16$16$1$1$1$0$0.001$0$-Inf$Inf$#DriveForceMax_N$32$16$1$1$1$0$100$0$-Inf$Inf$#DriveForceMin_N$48$16$1$1$1$0$100$0$-Inf$Inf$#  NSignals=4  IDPort=off  TimestampPort=off  ErrorPort=off  RemotePort=off  LengthPort=off  StatusPort=off  StartBits=str2num('[int32(0);int32(16);int32(32);int32(48)]')  SignalSizes=str2num('[int32(16);int32(16);int32(16);int32(16)]')  ByteOrders=str2num('[int32(1);int32(1);int32(1);int32(1)]')  DataTypes=str2num('[int32(1);int32(1);int32(1);int32(1)]')  MultiplexTypes=str2num('[int32(1);int32(1);int32(1);int32(1)]')  MultiplexValues=str2num('[double(0);double(0);double(0);double(0)]')  Factors=str2num('[double(0.001);double(0.001);double(100);double(100)]')  Offsets=str2num('[double(0);double(0);double(0);double(0)]')  Minimums=str2num('[double(-Inf);double(-Inf);double(-Inf);double(-Inf)]')  Maximums=str2num('[double(Inf);double(Inf);double(Inf);double(Inf)]')  ApplyMinMax=off
      settings: SourceProductName=Simulink Real-Time
  Terminator : Terminator
  While Iterator : WhileIterator  MaxIters=501  WhileBlockType=do-while
  omega_WheelFL_radps : Outport
  omega_WheelFR_radps : Outport  Port=2
  omega_WheelRL_radps : Outport  Port=3
  omega_WheelRR_radps : Outport  Port=4
  Out5 : Outport  Port=5
  x_Loc1_m : Outport  Port=6
  y_Loc1_m : Outport  Port=7
  Out8 : Outport  Port=8
  t_EstimateLoc1_s : Outport  Port=9
  Out10 : Outport  Port=10
  ax_CoGIMU1_mps2 : Outport  Port=11
  ay_CoGIMU1_mps2 : Outport  Port=12
  dPsi_YawRateIMU1_radps : Outport  Port=13
  Out14 : Outport  Port=14
  Hardware : Outport  Port=15
  AIDriver : Outport  Port=16
  ParkBrakeApplied_b : Outport  Port=17
  VehicleReady2Drive : Outport  Port=18
  SteeringAngleMax_rad : Outport  Port=19
  SteeringAngleMin_rad : Outport  Port=20
  DriveForceMax_N : Outport  Port=21
  DriveForceMin_N : Outport  Port=22
  wires:
  CAN Read/2 -> CAN Unpack/1, CAN Unpack2/1, CAN Unpack1/1, CAN Unpack3/1, CAN Unpack4/1
  CAN Unpack/4 -> omega_WheelRR_radps/1  "omega_WheelRR_radps"
  CAN Unpack2/2 -> y_Loc1_m/1  "y_Loc1_m"
  CAN Unpack2/5 -> Out10/1
  Input1/1 -> Terminator/1
  CAN Unpack/5 -> Out5/1
  CAN Read/1 -> While Iterator/1
  CAN Unpack1/1 -> ax_CoGIMU1_mps2/1  "ax_CoGIMU1_mps2"
  CAN Unpack2/4 -> t_EstimateLoc1_s/1  "t_EstimateLoc1_s"
  CAN Unpack2/3 -> Out8/1
  CAN Unpack/1 -> omega_WheelFL_radps/1  "omega_WheelFL_radps"
  CAN Unpack4/3 -> DriveForceMax_N/1  "DriveForceMax_N"
  CAN Unpack/3 -> omega_WheelRL_radps/1  "omega_WheelRL_radps"
  CAN Unpack1/2 -> ay_CoGIMU1_mps2/1  "ay_CoGIMU1_mps2"
  CAN Unpack4/2 -> SteeringAngleMin_rad/1  "SteeringAngleMin_rad"
  CAN Unpack3/2 -> AIDriver/1  "AIDriver"
  CAN Unpack3/3 -> ParkBrakeApplied_b/1  "ParkBrakeApplied_b"
  CAN Unpack1/4 -> Out14/1
  CAN Unpack4/1 -> SteeringAngleMax_rad/1  "SteeringAngleMax_rad"
  CAN Unpack/2 -> omega_WheelFR_radps/1  "omega_WheelFR_radps"
  CAN Unpack2/1 -> x_Loc1_m/1  "x_Loc1_m"
  CAN Unpack3/4 -> VehicleReady2Drive/1  "VehicleReady2Drive"
  CAN Unpack3/1 -> Hardware/1  "Hardware"
  CAN Unpack1/3 -> dPsi_YawRateIMU1_radps/1  "dPsi_YawRateIMU1_radps"
  CAN Unpack4/4 -> DriveForceMin_N/1  "DriveForceMin_N"

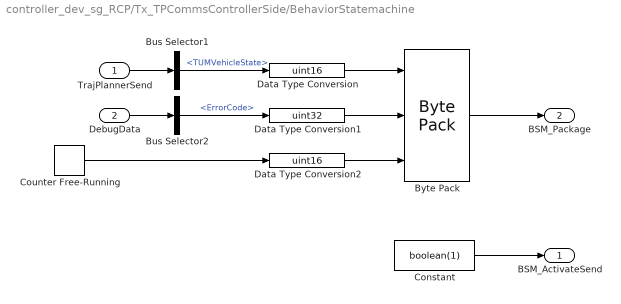
== system controller_dev_sg_RCP/Tx_TPCommsControllerSide/BehaviorStatemachine ==
  TrajPlannerSend : Inport
  DebugData : Inport  Port=2  OutDataTypeStr=Bus: mvdc_vehicle_dynamics_control_debug  PortDimensions=1
  Bus Selector1 : BusSelector  OutputSignals=TUMVehicleState
  Bus Selector2 : BusSelector  OutputSignals=ErrorCode
  Byte Pack : etargetslib/Byte Pack  datatypes={'uint16', 'uint32', 'uint16'}  byteAlign=1
  Constant : Constant  Value=boolean(1)  SampleTime=-1
  Counter Free-Running : simulink/Sources/Counter Free-Running  NumBits=8  tsamp=-1
  Data Type Conversion : DataTypeConversion  OutDataTypeStr=uint16
  Data Type Conversion1 : DataTypeConversion  OutDataTypeStr=uint32
  Data Type Conversion2 : DataTypeConversion  OutDataTypeStr=uint16
  BSM_ActivateSend : Outport
  BSM_Package : Outport  Port=2
  wires:
  Counter Free-Running/1 -> Data Type Conversion2/1
  Data Type Conversion/1 -> Byte Pack/1
  Data Type Conversion2/1 -> Byte Pack/3
  Byte Pack/1 -> BSM_Package/1
  Constant/1 -> BSM_ActivateSend/1
  TrajPlannerSend/1 -> Bus Selector1/1
  Bus Selector1/1 -> Data Type Conversion/1  "<TUMVehicleState>"
  DebugData/1 -> Bus Selector2/1
  Bus Selector2/1 -> Data Type Conversion1/1  "<ErrorCode>"
  Data Type Conversion1/1 -> Byte Pack/2

== system controller_dev_sg_RCP/Tx_TPCommsControllerSide/SendToBehaviorStatemachine1 ==
  Data : Inport
  Enable : EnablePort
  "Send " : xpcrtudplib/UDP Send  ipAddressVal=10.0.0.1  localPort=-1  toAddress=10.0.0.2  toPort=BehaviorStatemachineSend_Port  sampleTime=-1
      settings: SourceProductName=Simulink Real-Time  SourceProductBaseCode=XP
  Width : Width
  wires:
  Width/1 -> "Send "/2
  Data/1 -> Width/1, "Send "/1

== system controller_dev_sg_RCP/Tx_TPCommsControllerSide/SendToTrajectoryGeneration1 ==
  Data : Inport
  Enable : EnablePort
  "Send " : xpcrtudplib/UDP Send  ipAddressVal=10.0.0.1  localPort=-1  toAddress=10.0.0.2  toPort=TrajectoryGenerationSend_Port  sampleTime=-1
      settings: SourceProductName=Simulink Real-Time  SourceProductBaseCode=XP
  Width : Width
  wires:
  Width/1 -> "Send "/2
  Data/1 -> Width/1, "Send "/1

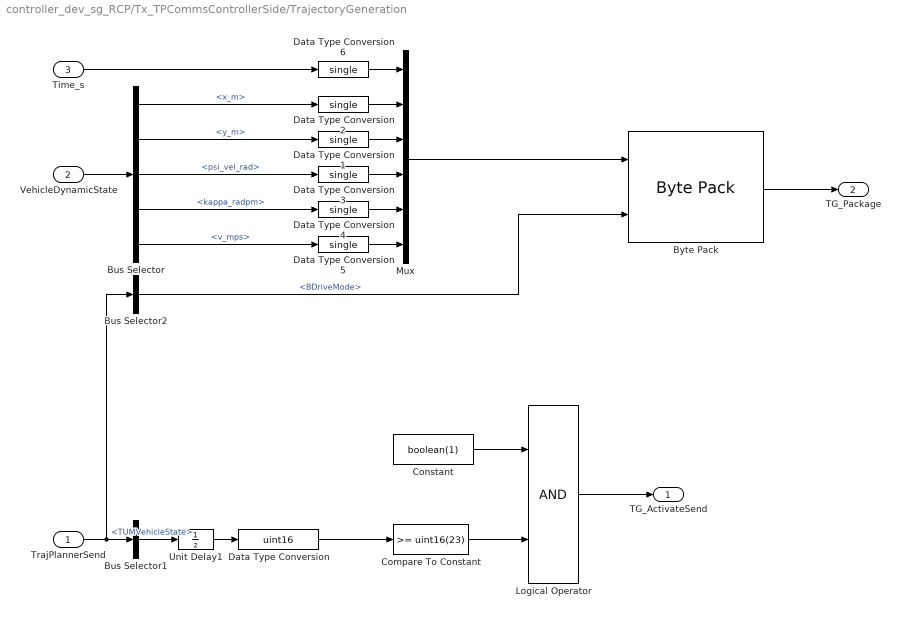
== system controller_dev_sg_RCP/Tx_TPCommsControllerSide/TrajectoryGeneration ==
  TrajPlannerSend : Inport
  VehicleDynamicState : Inport  Port=2
  Time_s : Inport  Port=3
  Bus Selector : BusSelector  OutputSignals=Pos.x_m,Pos.y_m,psi_vel_rad,kappa_radpm,v_mps
  Bus Selector1 : BusSelector  OutputSignals=TUMVehicleState
  Bus Selector2 : BusSelector  OutputSignals=BDriveMode
  Byte Pack : etargetslib/Byte Pack  datatypes={['single'], 'uint8'}  byteAlign=1
  Compare To Constant : simulink/Logic and Bit Operations/Compare To Constant  relop=>=  const=uint16(23)  OutDataTypeStr=boolean
  Constant : Constant  Value=boolean(1)  SampleTime=-1
  Data Type Conversion : DataTypeConversion  OutDataTypeStr=uint16
  Data Type Conversion{1..6} (6 alike) : DataTypeConversion  OutDataTypeStr=single
  Logical Operator : Logic  AllPortsSameDT=off  OutDataTypeStr=boolean
  Mux : Mux  Inputs=6
  Unit Delay1 : UnitDelay  InitialCondition=TUMVehicleState.OFF  SampleTime=tS
  TG_ActivateSend : Outport
  TG_Package : Outport  Port=2
  wires:
  Unit Delay1/1 -> Data Type Conversion/1
  Data Type Conversion/1 -> Compare To Constant/1
  Bus Selector/5 -> Data Type Conversion5/1  "<v_mps>"
  Data Type Conversion6/1 -> Mux/1
  Data Type Conversion4/1 -> Mux/5
  Data Type Conversion5/1 -> Mux/6
  Data Type Conversion1/1 -> Mux/3
  Data Type Conversion2/1 -> Mux/2
  Data Type Conversion3/1 -> Mux/4
  Time_s/1 -> Data Type Conversion6/1
  VehicleDynamicState/1 -> Bus Selector/1
  Mux/1 -> Byte Pack/1
  Bus Selector/4 -> Data Type Conversion4/1  "<kappa_radpm>"
  Byte Pack/1 -> TG_Package/1
  Bus Selector/1 -> Data Type Conversion2/1  "<x_m>"
  Bus Selector/2 -> Data Type Conversion1/1  "<y_m>"
  Bus Selector/3 -> Data Type Conversion3/1  "<psi_vel_rad>"
  Compare To Constant/1 -> Logical Operator/2
  Logical Operator/1 -> TG_ActivateSend/1
  Constant/1 -> Logical Operator/1
  TrajPlannerSend/1 -> Bus Selector2/1, Bus Selector1/1
  Bus Selector1/1 -> Unit Delay1/1  "<TUMVehicleState>"
  Bus Selector2/1 -> Byte Pack/2  "<BDriveMode>"

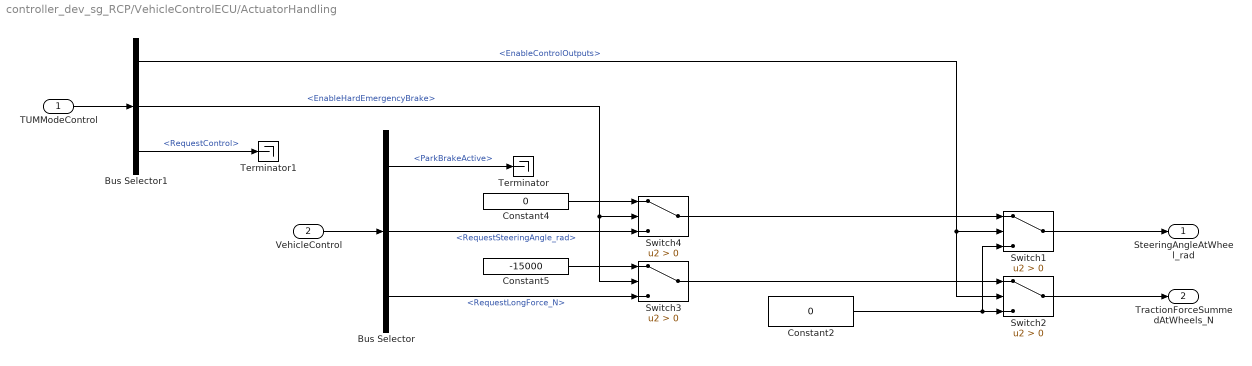
== system controller_dev_sg_RCP/VehicleControlECU/ActuatorHandling ==
  TUMModeControl : Inport  OutDataTypeStr=Bus: TUMModeControl
  VehicleControl : Inport  Port=2  OutDataTypeStr=Bus: VehicleControl
  Bus Selector : BusSelector  OutputSignals=ParkBrakeActive,RequestSteeringAngle_rad,RequestLongForce_N
  Bus Selector1 : BusSelector  OutputSignals=EnableControlOutputs,EnableHardEmergencyBrake,RequestControl
  Constant2 : Constant  Value=0
  Constant4 : Constant  Value=0
  Constant5 : Constant  Value=-15000
  Switch{1..4} (4 alike) : Switch  Criteria=u2 > Threshold
  Terminator : Terminator
  Terminator1 : Terminator
  SteeringAngleAtWheel_rad : Outport
  TractionForceSummedAtWheels_N : Outport  Port=2
  wires:
  Bus Selector1/1 -> Switch2/2, Switch1/2  "<EnableControlOutputs>"
  TUMModeControl/1 -> Bus Selector1/1
  Bus Selector/3 -> Switch3/3  "<RequestLongForce_N>"
  Constant2/1 -> Switch1/3, Switch2/3
  VehicleControl/1 -> Bus Selector/1
  Bus Selector/2 -> Switch4/3  "<RequestSteeringAngle_rad>"
  Constant4/1 -> Switch4/1
  Constant5/1 -> Switch3/1
  Bus Selector1/2 -> Switch3/2, Switch4/2  "<EnableHardEmergencyBrake>"
  Bus Selector/1 -> Terminator/1  "<ParkBrakeActive>"
  Bus Selector1/3 -> Terminator1/1  "<RequestControl>"
  Switch4/1 -> Switch1/1
  Switch3/1 -> Switch2/1
  Switch1/1 -> SteeringAngleAtWheel_rad/1
  Switch2/1 -> TractionForceSummedAtWheels_N/1
